simulink library "realisticSensors_cl"  (R2022a)
settings: Solver=VariableStepAuto  StartTime=0.0  StopTime=10.0  RelTol=1e-3
undefined symbols (not defined in the file or in its folder): initializeBussesFromBlock
libraries: lasPosEst_cl x1, lineAngleSensor x1, lineAngleSensorObserver x1
settings Model: Creator=mcobb  LastModifiedBy=lhill8
settings SolverCC: AlgebraicLoopSolver=TrustRegion
settings DebuggingCC: UnconnectedInputMsg=warning  UnconnectedOutputMsg=warning  UnconnectedLineMsg=warning  SFMachineParentedDataDiag=warning  ArithmeticOperatorsInVariantConditions=warning
settings SFSimCC: CustomCodeUndefinedFunction=UseInterfaceOnly

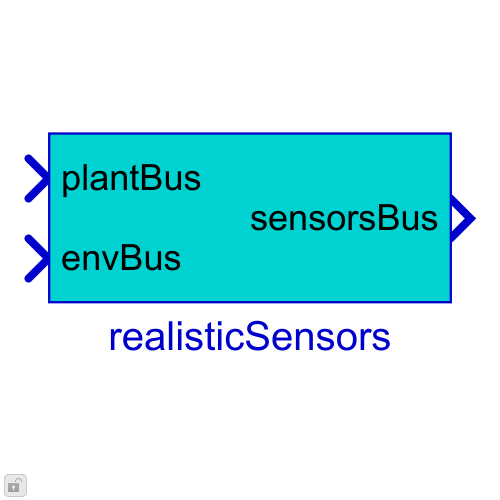
[thumbnail: Simulink's stored preview of the top-level diagram]
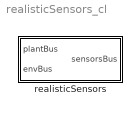
== system realisticSensors_cl ==
  realisticSensors : Subsystem  LoadFcn=initializeBussesFromBlock(gcb)  InitFcn=initializeBussesFromBlock(gcb)  StartFcn=initializeBussesFromBlock(gcb)  VariantControl=VSS_sensors_realisticSensors

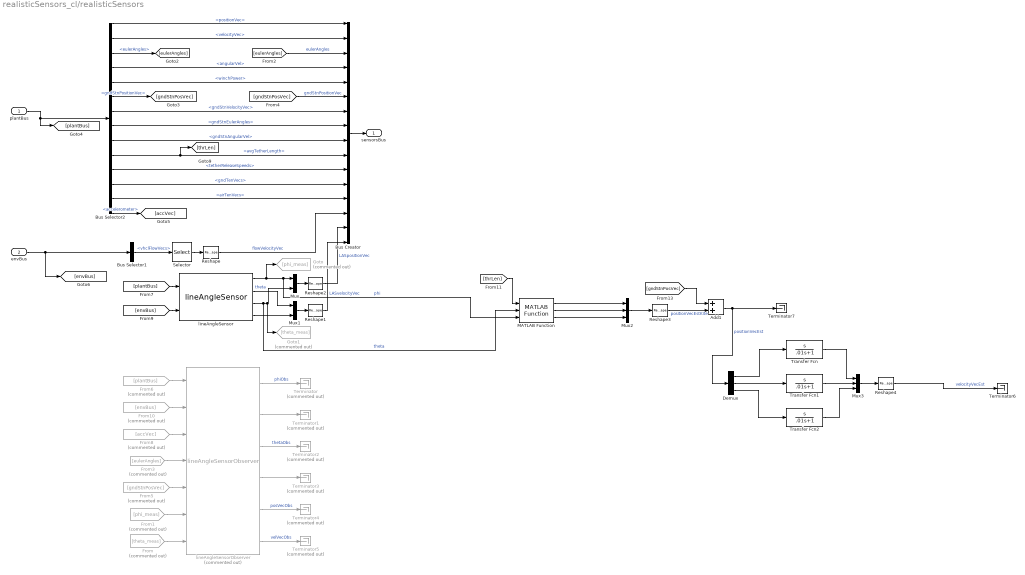
== system realisticSensors_cl/realisticSensors ==
  plantBus : Inport  OutDataTypeStr=Bus: plantBus
  envBus : Inport  Port=2  OutDataTypeStr=Bus: envBus
  Add1 : Sum
  Bus Creator : BusCreator  Inputs=16
  Bus Selector1 : BusSelector  OutputSignals=vhclFlowVecs
  Bus Selector2 : BusSelector  OutputSignals=positionVec,velocityVec,eulerAngles,angularVel,winchPower,gndStnPositionVec,gndStnVelocityVec,gndStnEulerAngles,gndStnAngularVel,avgTetherLength,tetherReleaseSpeeds,gndTenVecs,airTenVecs,accelerometer
  Demux : Demux  Outputs=3
  From : From  Commented=on  GotoTag=theta_meas
  From1 : From  Commented=on  GotoTag=phi_meas
  From10 : From  Commented=on  GotoTag=envBus
  From3 : From  Commented=on  GotoTag=eulerAngles
  From5 : From  Commented=on  GotoTag=gndStnPosVec
  From6 : From  Commented=on  GotoTag=plantBus
  From8 : From  Commented=on  GotoTag=accVec
  Goto : Goto  Commented=on  GotoTag=phi_meas
  Goto1 : Goto  Commented=on  GotoTag=theta_meas
  MATLAB Function : lasPosEst_cl/lasPosEst/MATLAB Function  SystemSampleTime=-1  VariantActivationTime=update diagram  Latency=0  AutoFrameSizeCalculation=off
  Mux : Mux  Inputs=2
  Mux1 : Mux  Inputs=2
  Mux2 : Mux  Inputs=3
  Mux3 : Mux  Inputs=3
  Reshape{,1..4} (5 alike) : Reshape  OutputDimensionality=Column vector (2-D)
  Selector : Selector  NumberOfDimensions=2  InputPortWidth=3  IndexOptions=Select all,Index vector (dialog)  Indices=[1 3],1  OutputSizes=1,1
  Terminator{,1..5} (6 alike) : Terminator  Commented=on
  Terminator6 : Terminator
  Terminator7 : Terminator
  Transfer Fcn : TransferFcn  Numerator=[1 0]  Denominator=[.01 1]
  Transfer Fcn1 : TransferFcn  Numerator=[1 0]  Denominator=[.01 1]
  Transfer Fcn2 : TransferFcn  Numerator=[1 0]  Denominator=[.01 1]
  lineAngleSensor : lineAngleSensor/lineAngleSensor  las=las  env=env
  lineAngleSensorObserver : lineAngleSensorObserver/lineAngleSensorObserver  Commented=on  las=las  env=env
  sensorsBus : Outport  OutDataTypeStr=Bus: sensorsBus  VectorParamsAs1DForOutWhenUnconnected=off
  wires:
  Bus Selector2/8 -> Bus Creator/8  "<gndStnEulerAngles>"
  Bus Selector2/4 -> Bus Creator/4  "<angularVel>"
  Bus Selector2/3 -> [eulerAngles]  "<eulerAngles>"
  Bus Selector2/9 -> Bus Creator/9  "<gndStnAngularVel>"
  Bus Creator/1 -> sensorsBus/1
  Bus Selector2/12 -> Bus Creator/12  "<gndTenVecs>"
  Bus Selector2/7 -> Bus Creator/7  "<gndStnVelocityVec>"
  Bus Selector2/10 -> [thrLen], Bus Creator/10  "<avgTetherLength>"
  Bus Selector2/11 -> Bus Creator/11  "<tetherReleaseSpeeds>"
  envBus/1 -> [envBus], Bus Selector1/1
  Mux1/1 -> Reshape1/1
  Mux/1 -> Reshape2/1
  lineAngleSensor/3 -> MATLAB Function/2, Goto1/1, Mux/2  "theta"
  Selector/1 -> Reshape/1
  Reshape1/1 -> Bus Creator/16  "LASvelocityVec"
  Bus Selector2/2 -> Bus Creator/2  "<velocityVec>"
  lineAngleSensor/4 -> Mux1/2
  Bus Selector2/5 -> Bus Creator/5  "<winchPower>"
  Bus Selector2/1 -> Bus Creator/1  "<positionVec>"
  Bus Selector1/1 -> Selector/1  "<vhclFlowVecs>"
  Reshape/1 -> Bus Creator/14  "flowVelocityVec"
  Reshape2/1 -> Bus Creator/15  "LASpositionVec"
  Bus Selector2/6 -> [gndStnPosVec]  "<gndStnPositionVec>"
  From/1 -> lineAngleSensorObserver/7
  From1/1 -> lineAngleSensorObserver/6
  lineAngleSensorObserver/1 -> Terminator/1  "phiObs"
  lineAngleSensorObserver/2 -> Terminator1/1
  lineAngleSensorObserver/3 -> Terminator2/1  "thetaObs"
  lineAngleSensorObserver/4 -> Terminator3/1
  lineAngleSensorObserver/5 -> Terminator4/1  "posVecObs"
  lineAngleSensorObserver/6 -> Terminator5/1  "velVecObs"
  [eulerAngles] -> Bus Creator/3  "eulerAngles"
  From3/1 -> lineAngleSensorObserver/4
  [gndStnPosVec] -> Bus Creator/6  "gndStnPositionVec"
  From5/1 -> lineAngleSensorObserver/5
  plantBus/1 -> [plantBus], Bus Selector2/1
  From6/1 -> lineAngleSensorObserver/1
  [plantBus] -> lineAngleSensor/1
  Bus Selector2/14 -> [accVec]  "<accelerometer>"
  From8/1 -> lineAngleSensorObserver/3
  [envBus] -> lineAngleSensor/2
  From10/1 -> lineAngleSensorObserver/2
  Bus Selector2/13 -> Bus Creator/13  "<airTenVecs>"
  lineAngleSensor/2 -> Mux1/1  "theta"
  Mux2/1 -> Reshape3/1
  [thrLen] -> MATLAB Function/1
  Transfer Fcn1/1 -> Mux3/2
  lineAngleSensor/1 -> Goto/1, MATLAB Function/3, Mux/1  "phi"
  Transfer Fcn2/1 -> Mux3/3
  Demux/1 -> Transfer Fcn/1
  Demux/3 -> Transfer Fcn2/1
  Mux3/1 -> Reshape4/1
  MATLAB Function/3 -> Mux2/3
  Reshape3/1 -> Add1/2  "positionVecEstKite"
  [gndStnPosVec] -> Add1/1
  Add1/1 -> Terminator7/1, Demux/1  "positionVecEst"
  Demux/2 -> Transfer Fcn1/1
  Transfer Fcn/1 -> Mux3/1
  MATLAB Function/1 -> Mux2/1
  Reshape4/1 -> Terminator6/1  "velocityVecEst"
  MATLAB Function/2 -> Mux2/2
